simulink model "AOO_wRequirementsTable"  (R2022a)
settings: Solver=FixedStepAuto  StartTime=0.0  StopTime=0.59  FixedStep=1e-4  RelTol=1e-3  EnableMultiTasking=on
undefined symbols (not defined in the file): D10, D11, D2, D4, D5, D8, D9, PTA0, PTA2, PTB23, PTB9, PTC4, PTD0, PTD2
libraries: frdmk64flib x7
settings Model: ExtModeTrigDuration=5  Creator=kemij  LastModifiedBy=bmile
settings OptimizationCC: EnhancedBackFolding=on  PassReuseOutputArgsAs=Individual arguments  ZeroExternalMemoryAtStartup=off  ZeroInternalMemoryAtStartup=off  MaxStackSize=64  OptimizeBlockOrder=speed  DifferentSizesBufferReuse=on  OptimizationCustomize=off  EfficientTunableParamExpr=on
settings DebuggingCC: ParameterTunabilityLossMsg=error
settings HardwareCC: ProdBitPerPointer=32  ProdBitPerSizeT=32  ProdBitPerPtrDiffT=32  ProdLargestAtomicInteger=Long  ProdLargestAtomicFloat=Double  ProdWordSize=32  ProdHWDeviceType=ARM Compatible->ARM Cortex
settings SFSimCC: MATLABDynamicMemAlloc=off
settings RTWCC: SystemTargetFile=ert.tlc  HardwareBoard=NXP FRDM-K64F  TLCOptions="-aInlineSetEventsForThisBaseRateFcn=TLC_FALSE -aSuppressMultiTaskScheduler=TLC_FALSE  -aRateBasedStepFcn=0"  TemplateMakefile=ert_default_tmf  Toolchain=GNU Tools for ARM Embedded Processors
settings CodeAppCC: ForceParamTrailComments=on  IgnoreCustomStorageClasses=off  OperatorAnnotations=on  SimulinkDataObjDesc=on  SFDataObjDesc=on  InsertBlockDesc=on
settings ERTTargetCC: ExtModeTransport=4  ExtModeMexFile=sendToCommService

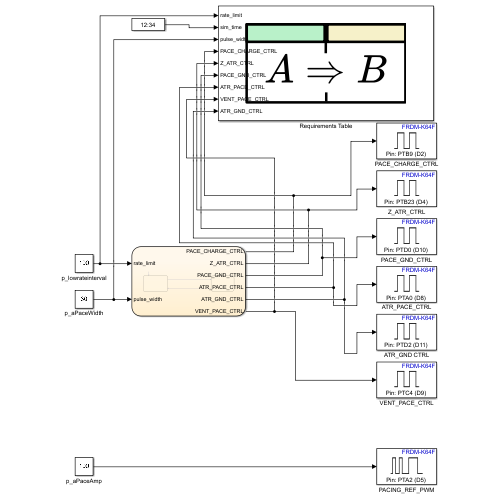
[thumbnail: Simulink's stored preview of the top-level diagram]
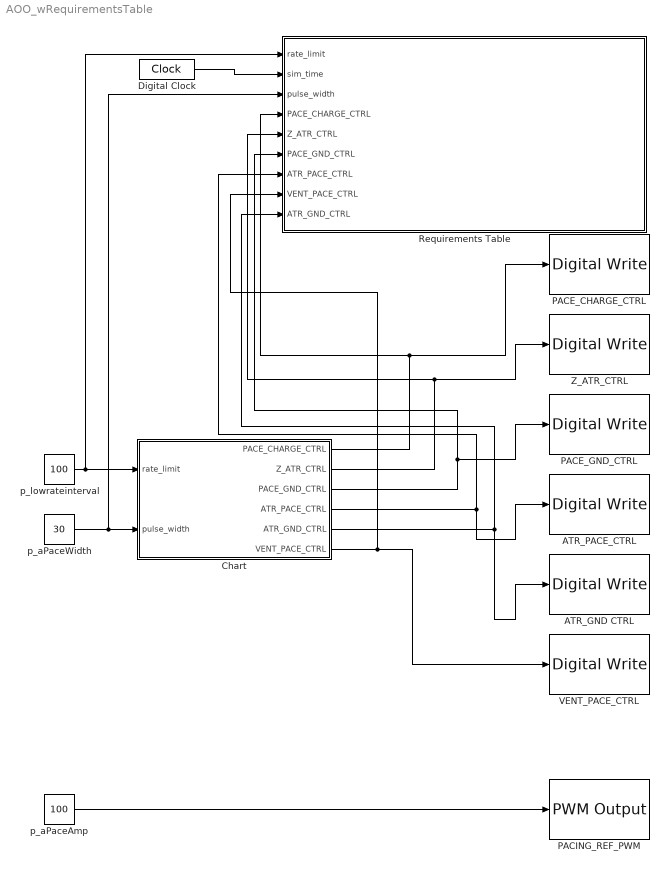
== system AOO_wRequirementsTable ==
  ATR_GND CTRL : frdmk64flib/Digital Write  Whichpin=PTD2 (D11)
  ATR_PACE_CTRL : frdmk64flib/Digital Write  Whichpin=PTA0 (D8)
  Chart : Stateflow chart  TreatAsAtomicUnit=on
  Digital Clock : DigitalClock  SampleTime=0.0001
  PACE_CHARGE_CTRL : frdmk64flib/Digital Write  Whichpin=PTB9 (D2)
  PACE_GND_CTRL : frdmk64flib/Digital Write  Whichpin=PTD0 (D10)
  PACING_REF_PWM : frdmk64flib/PWM Output  Whichpin=PTA2 (D5)  InitialFrequency=2000  InitialDutyCycle=0
  Requirements Table : Requirements Table  TreatAsAtomicUnit=on
  VENT_PACE_CTRL : frdmk64flib/Digital Write  Whichpin=PTC4 (D9)
  Z_ATR_CTRL : frdmk64flib/Digital Write  Whichpin=PTB23 (D4)
  p_aPaceAmp : Constant  Value=100
  p_aPaceWidth : Constant  Value=30
  p_lowrateinterval : Constant  Value=100
  wires:
  p_aPaceAmp/1 -> PACING_REF_PWM/1
  Chart/5(ATR_GND_CTRL) -> ATR_GND CTRL/1, Requirements Table/9(ATR_GND_CTRL)
  Chart/3(PACE_GND_CTRL) -> PACE_GND_CTRL/1, Requirements Table/6(PACE_GND_CTRL)
  Chart/2(Z_ATR_CTRL) -> Z_ATR_CTRL/1, Requirements Table/5(Z_ATR_CTRL)
  p_aPaceWidth/1 -> Requirements Table/3(pulse_width), Chart/2(pulse_width)
  p_lowrateinterval/1 -> Chart/1(rate_limit), Requirements Table/1(rate_limit)
  Chart/1(PACE_CHARGE_CTRL) -> PACE_CHARGE_CTRL/1, Requirements Table/4(PACE_CHARGE_CTRL)
  Chart/4(ATR_PACE_CTRL) -> ATR_PACE_CTRL/1, Requirements Table/7(ATR_PACE_CTRL)
  Digital Clock/1 -> Requirements Table/2(sim_time)
  Chart/6(VENT_PACE_CTRL) -> Requirements Table/8(VENT_PACE_CTRL), VENT_PACE_CTRL/1

== stateflow chart AOO_wRequirementsTable/Chart ==
  state Charging_Discharging
    entry:
    ATR_PACE_CTRL = false
    VENT_PACE_CTRL=false
    PACE_CHARGE_CTRL = true
    ATR_GND_CTRL = true
    PACE_GND_CTRL = true
    Z_ATR_CTRL=false
  state Pace_Heart
    entry:
    ATR_PACE_CTRL = true
    PACE_CHARGE_CTRL = false
    PACE_GND_CTRL = true
    ATR_GND_CTRL = false
    ATR_GND_CTRL = false
  (default) -> Charging_Discharging
  Charging_Discharging -> Pace_Heart : after(((1/rate_limit)*60000)-pulse_width,msec)
  Pace_Heart -> Charging_Discharging : after(pulse_width,msec)
  data: rate_limit input; pulse_width input; PACE_CHARGE_CTRL output boolean; Z_ATR_CTRL output boolean; PACE_GND_CTRL output boolean; ATR_PACE_CTRL output boolean; ATR_GND_CTRL output boolean; VENT_PACE_CTRL output

== stateflow chart AOO_wRequirementsTable/Requirements Table ==
  (default) -> (junction 1073743090)
  (junction 1073743090) -> (junction 1073743091) : {
      | % SF_REQ_REV_07
      | }
  (junction 1073743091) -> (junction 1073743093) : {
      | % HEADER_ASSIGNMENTS
      |
      | }
  (junction 1073743093) -> (junction 1073743095) : {
      | % START_A_4
      | }
  (junction 1073743095) -> (junction 1073743097) : {
      | }
  (junction 1073743097) -> (junction 1073743099)
  (junction 1073743099) -> (junction 1073743101) : {
      | }
  (junction 1073743101) -> (junction 1073743103) : {
      | % END_A_4
      | }
  (junction 1073743103) -> (junction 1073743206) : {
      | % START_R_1
      | }
  (junction 1073743206) -> (junction 1073743208) : {
      | }
  (junction 1073743208) -> (junction 1073743210)
  (junction 1073743210) -> (junction 1073743212) [order 1] : [(((sim_time) >= (0) && (sim_time) <= (((1/rate_limit)*60)-(pulse_width/1000))))]
  (junction 1073743210) -> (junction 1073743218) [order 2]
  (junction 1073743212) -> (junction 1073743214) : {
      | reqtable_postcondition((((ATR_PACE_CTRL) == (false))) && (((VENT_PACE_CTRL) == (false))) && (((PACE_CHARGE_CTRL) == (true))) && (((ATR_GND_CTRL) == (true))) && (((PACE_GND_CTRL) == (true))) && (((Z_ATR_CTRL) == (false))), 'R:1');
      |
      |
      | }
  (junction 1073743214) -> (junction 1073743216) : {
      | }
  (junction 1073743216) -> (junction 1073743218)
  (junction 1073743218) -> (junction 1073743220)
  (junction 1073743220) -> (junction 1073743222) : {
      | % END_R_1
      | }
  (junction 1073743222) -> (junction 1073743123) : {
      | % START_R_7
      | }
  (junction 1073743123) -> (junction 1073743125) : {
      | }
  (junction 1073743125) -> (junction 1073743127)
  (junction 1073743127) -> (junction 1073743129) [order 1] : [(((sim_time) > (((1/rate_limit)*60)-(pulse_width/1000)) && (sim_time) < (((1/rate_limit)*60)+(pulse_width/1000))))]
  (junction 1073743127) -> (junction 1073743135) [order 2]
  (junction 1073743129) -> (junction 1073743131) : {
      | reqtable_postcondition((((ATR_PACE_CTRL) == (true))) && (((VENT_PACE_CTRL) == (false))) && (((PACE_CHARGE_CTRL) == (false))) && (((ATR_GND_CTRL) == (false))) && (((PACE_GND_CTRL) == (true))) && (((Z_ATR_CTRL) == (false))), 'R:2');
      |
      |
      | }
  (junction 1073743131) -> (junction 1073743133) : {
      | }
  (junction 1073743133) -> (junction 1073743135)
  (junction 1073743135) -> (junction 1073743137)
  (junction 1073743137) -> (junction 1073743139) : {
      | % END_R_7
      | }
  data: rate_limit input; sim_time input; pulse_width input; PACE_CHARGE_CTRL input; Z_ATR_CTRL input; PACE_GND_CTRL input; ATR_PACE_CTRL input; VENT_PACE_CTRL input; ATR_GND_CTRL input
